simulink model "model_testing"  (R2022b)
settings: Solver=VariableStepAuto  StartTime=0.0  StopTime=1  RelTol=1e-6
values from neighbouring files (symbols this model uses):
  A = d*A1 + dp*A2    [Final_project.m]    (also in SSA.m; ssa_2.m = inv(K)*A)
  B = d*B1 + dp*B2    [Final_project.m]    (also in SSA.m; ssa_2.m = inv(K)*B_ss)
  C = d*C1 + dp*C2    [Final_project.m]    (also in SSA.m; ssa_2.m = 6e-06)
  D = d*D1 + dp*D2    [Final_project.m]    (also in SSA.m; ssa_2.m = D_ss)
  Vd = 0.9    [ssa_2.m]
  Vi = 50    [ssa_2.m]
settings Model: Creator=maxim  LastModifiedBy=maxim

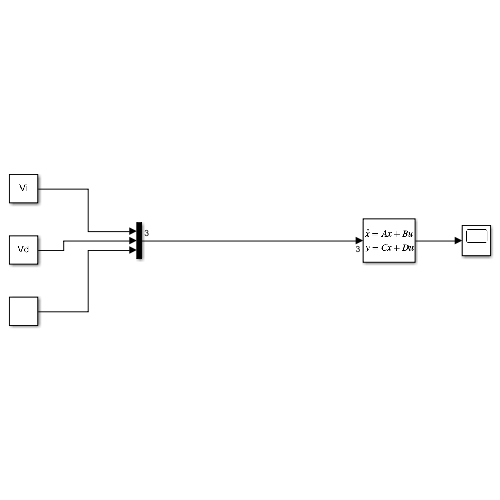
[thumbnail: Simulink's stored preview of the top-level diagram]
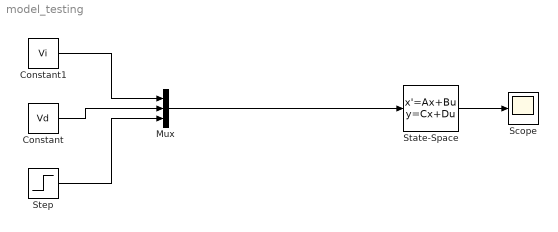
== system model_testing ==
  Constant : Constant  Value=Vd
  Constant1 : Constant  Value=Vi
  Mux : Mux  Inputs=3
  Scope : Scope
  State-Space : StateSpace  A=A  B=B  C=C  D=D  InitialCondition=0
  Step : Step  Time=0.1  After=0.01  SampleTime=0
  wires:
  State-Space/1 -> Scope/1
  Constant/1 -> Mux/2
  Constant1/1 -> Mux/1
  Step/1 -> Mux/3
  Mux/1 -> State-Space/1
